simulink library "pmm"  (R2021b)
settings: Solver=VariableStepAuto  StartTime=0.0  StopTime=10.0  RelTol=1e-3
undefined symbols (not defined in the file): APMM_CoolgFanActCurr_X_pct, APMM_EWP1Curr_X_c, APMM_EWP3Curr_X_c, APMM_LVBattChktime_X_enum, APMM_LVBattChrgtime_X_enum, APMM_LVChrgLv_X_mV, ENUM_ANTITHEFT_ALARM, ENUM_ANTITHEFT_ARM, ENUM_ANTITHEFT_DISARM, ENUM_ANTITHEFT_WAIT, ENUM_APSSYSTEMSTA_REMOTEACTIVE, ENUM_CHRGPLUGSTA_NONE, ENUM_CRASHSTATE_FRONTFIRSTLV, ENUM_CRASHSTATE_LEFTSIDE, ENUM_CRASHSTATE_RIGHTSIDE, ENUM_DRIVETRAIN_AWD, ENUM_DRIVETRAIN_FWD, ENUM_DRIVETRAIN_RWD, ENUM_DRSEATSTA_EMPTY, ENUM_DRSEATSTA_INVALID, ENUM_DRSEATSTA_OCCUPIED, ENUM_EPBSTA_APPLIED, ENUM_GEARACTUALPOSN_D, ENUM_GEARACTUALPOSN_N, ENUM_GEARACTUALPOSN_P, ENUM_GEARACTUALPOSN_R, ENUM_HVBATTREADYPRE_READY, ENUM_OTACHKSTA_NOREQUEST, ENUM_OTACHKSTA_NOTIMEOUT, ENUM_OTACHKSTA_TIMEOUT, ENUM_PDKEYRAWLULOCK_INLOCK, ENUM_PDKEYRAWLULOCK_INUNLOCK, ENUM_PDKEYRAWPS_INPS, ENUM_PDKEYSTA_LOCK, ENUM_PDKEYSTA_PS, ENUM_PDKEYSTA_UNAVALIABLE, ENUM_PDKEYSTA_UNLOCK, ENUM_POWERSTA_OFF, ENUM_POWERSTA_OFFC, ENUM_POWERSTA_STANDBY, ENUM_PWRREQOTA_NOREQUEST, ENUM_PWRREQOTA_REQPOWEROFF, ENUM_PWRREQOTA_REQPOWERSTDBY, ENUM_PWRSTASW_READY, ENUM_V2LSTA_NOPLUG, ENUM_VEHICLETYPE_D31L24, ENUM_VEHMALFUNLEVEL_LEVEL3, ENUM_VEHMALFUNLEVEL_LEVEL4, FALSE, KPMM_AllDoorClosedHoldTime_s, KPMM_APSAllowThd_pct, KPMM_BattDownFailtime_s, KPMM_BattUpFailtime_s, KPMM_BattUpResetRty_cnt, KPMM_BattUpResetSW_flg, KPMM_BattUpResetTO_s, KPMM_BattUpRstDlyTO_s, KPMM_BrakeSWHoldTime_s, KPMM_CANValidChkFailtime_s, KPMM_ChrgPlugHoldTime_s ... (+87)
libraries: simulink x29, hcu_lib x24
(part 3 of 7)

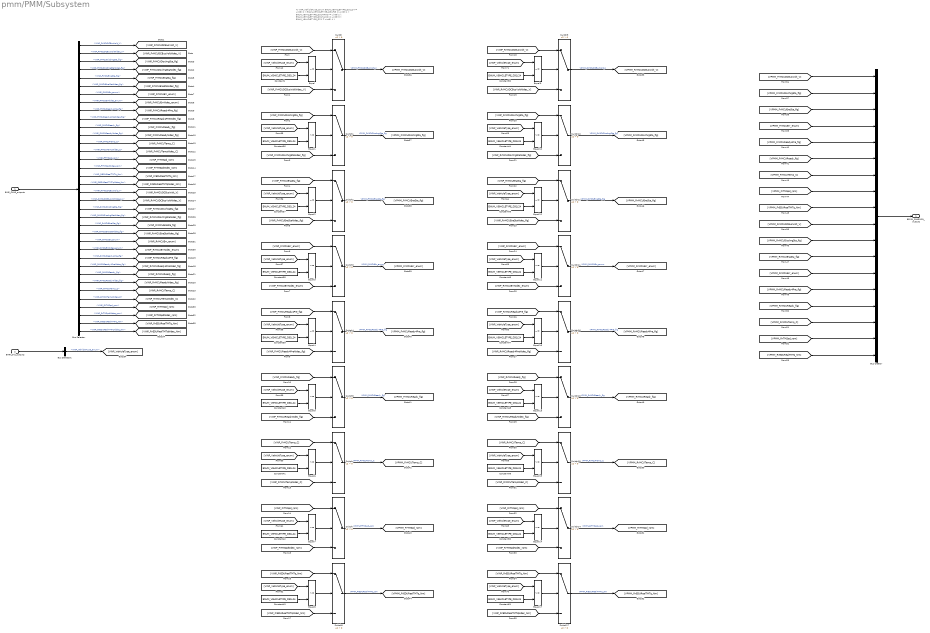
== system pmm/PMM/Subsystem ==
  note: % VINP_VehicleType_enum
      | ENUM_VEHICLETYPE_D31L24         	= uint8(  0  );
      | ENUM_VEHICLETYPE_D31F25         	= uint8(  1  );
      | ENUM_VEHICLETYPE_D31HRWD        = uint8(  2  );
      | ENUM_VEHICLETYPE_D31HAWD        = uint8(  3  );
      | ENUM_VEHICLETYPE_D21           		= uint8(  4  );
  BINP_CAN3_outputs : Inport
  BINP_SYS_outputs : Inport  Port=2
  Bus Creator : BusCreator  Inputs=18
  Bus Selector : BusSelector  OutputSignals=VINP_FrMCUDCBusVolt_V,VINP_FrMCUDCBusVoltNidec_V,VINP_FrMCUDischrgSta_flg,VINP_FrMCUDischrgStaNidec_flg,VINP_FrMCUEnaSta_flg,VINP_FrMCUEnaStaNidec_flg,VINP_FrMCUErr_enum,VINP_FrMCUErrNidec_enum,VINP_FrMCUReady4Pre_flg,VINP_FrMCUReady4PreNidec_flg,VINP_FrMCUReady_flg,VINP_FrMCUReadyNidec_flg,VINP_FrMCUTemp_C,VINP_FrMCUTempNidec_C,VINP_FrTMSpd_rpm,VINP_FrTMSpdNidec_rpm,VINP_FrEDURealTMTq_Nm,VINP_FrEDURealTMTqNidec_Nm,VINP_RrMCUDCBusVolt_V,VINP_RrMCUDCBusVoltNidec_V,VINP_RrMCUDischrgSta_flg,VINP_RrMCUDischrgStaNidec_flg,VINP_RrMCUEnaSta_flg,VINP_RrMCUEnaStaNidec_flg,VINP_RrMCUErr_enum,VINP_RrMCUErrNidec_enum,VINP_RrMCUReady4Pre_flg,VINP_RrMCUReady4PreNidec_flg,VINP_RrMCUReady_flg,VINP_RrMCUReadyNidec_flg,VINP_RrMCUTemp_C,VINP_RrMCUTempNidec_C,VINP_RrTMSpd_rpm,VINP_RrTMSpdNidec_rpm,VINP_RrEDURealTMTq_Nm,VINP_RrEDURealTMTqNidec_Nm
  Bus Selector1 : BusSelector  OutputSignals=VINP_VehicleType_enum
  Constant{1,36..52} (18 alike) : Constant  Value=ENUM_VEHICLETYPE_D31L24
  Equal{,1..17} (18 alike) : RelationalOperator  Operator=~=  OutDataTypeStr=boolean  RndMeth=Simplest
  Switch{,1..17} (18 alike) : Switch  Criteria=u2 > Threshold
  BPMM_CAN3MCU_outputs : Outport
  wires:
  BINP_CAN3_outputs/1 -> Bus Selector/1
  Bus Selector/1 -> [VINP_FrMCUDCBusVolt_V]  "<VINP_FrMCUDCBusVolt_V>"
  Bus Selector/2 -> [VINP_FrMCUDCBusVoltNidec_V]  "<VINP_FrMCUDCBusVoltNidec_V>"
  Bus Selector/3 -> [VINP_FrMCUDischrgSta_flg]  "<VINP_FrMCUDischrgSta_flg>"
  Bus Selector/4 -> [VINP_FrMCUDischrgStaNidec_flg]  "<VINP_FrMCUDischrgStaNidec_flg>"
  Bus Selector/5 -> [VINP_FrMCUEnaSta_flg]  "<VINP_FrMCUEnaSta_flg>"
  Bus Selector/6 -> [VINP_FrMCUEnaStaNidec_flg]  "<VINP_FrMCUEnaStaNidec_flg>"
  Bus Selector/7 -> [VINP_FrMCUErr_enum]  "<VINP_FrMCUErr_enum>"
  Bus Selector/8 -> [VINP_FrMCUErrNidec_enum]  "<VINP_FrMCUErrNidec_enum>"
  Bus Selector/9 -> [VINP_FrMCUReady4Pre_flg]  "<VINP_FrMCUReady4Pre_flg>"
  Bus Selector/10 -> [VINP_FrMCUReady4PreNidec_flg]  "<VINP_FrMCUReady4PreNidec_flg>"
  Bus Selector/11 -> [VINP_FrMCUReady_flg]  "<VINP_FrMCUReady_flg>"
  Bus Selector/12 -> [VINP_FrMCUReadyNidec_flg]  "<VINP_FrMCUReadyNidec_flg>"
  Bus Selector/13 -> [VINP_FrMCUTemp_C]  "<VINP_FrMCUTemp_C>"
  Bus Selector/14 -> [VINP_FrMCUTempNidec_C]  "<VINP_FrMCUTempNidec_C>"
  Bus Selector/15 -> [VINP_FrTMSpd_rpm]  "<VINP_FrTMSpd_rpm>"
  Bus Selector/16 -> [VINP_FrTMSpdNidec_rpm]  "<VINP_FrTMSpdNidec_rpm>"
  Bus Selector/17 -> [VINP_FrEDURealTMTq_Nm]  "<VINP_FrEDURealTMTq_Nm>"
  Bus Selector/18 -> [VINP_FrEDURealTMTqNidec_Nm]  "<VINP_FrEDURealTMTqNidec_Nm>"
  Bus Selector/19 -> [VINP_RrMCUDCBusVolt_V]  "<VINP_RrMCUDCBusVolt_V>"
  Bus Selector/20 -> [VINP_RrMCUDCBusVoltNidec_V]  "<VINP_RrMCUDCBusVoltNidec_V>"
  Bus Selector/21 -> [VINP_RrMCUDischrgSta_flg]  "<VINP_RrMCUDischrgSta_flg>"
  Bus Selector/22 -> [VINP_RrMCUDischrgStaNidec_flg]  "<VINP_RrMCUDischrgStaNidec_flg>"
  Bus Selector/23 -> [VINP_RrMCUEnaSta_flg]  "<VINP_RrMCUEnaSta_flg>"
  Bus Selector/24 -> [VINP_RrMCUEnaStaNidec_flg]  "<VINP_RrMCUEnaStaNidec_flg>"
  Bus Selector/25 -> [VINP_RrMCUErr_enum]  "<VINP_RrMCUErr_enum>"
  Bus Selector/26 -> [VINP_RrMCUErrNidec_enum]  "<VINP_RrMCUErrNidec_enum>"
  Bus Selector/27 -> [VINP_RrMCUReady4Pre_flg]  "<VINP_RrMCUReady4Pre_flg>"
  Bus Selector/28 -> [VINP_RrMCUReady4PreNidec_flg]  "<VINP_RrMCUReady4PreNidec_flg>"
  Bus Selector/29 -> [VINP_RrMCUReady_flg]  "<VINP_RrMCUReady_flg>"
  Bus Selector/30 -> [VINP_RrMCUReadyNidec_flg]  "<VINP_RrMCUReadyNidec_flg>"
  Bus Selector/31 -> [VINP_RrMCUTemp_C]  "<VINP_RrMCUTemp_C>"
  Bus Selector/32 -> [VINP_RrMCUTempNidec_C]  "<VINP_RrMCUTempNidec_C>"
  Bus Selector/33 -> [VINP_RrTMSpd_rpm]  "<VINP_RrTMSpd_rpm>"
  Bus Selector/34 -> [VINP_RrTMSpdNidec_rpm]  "<VINP_RrTMSpdNidec_rpm>"
  Bus Selector/35 -> [VINP_RrEDURealTMTq_Nm]  "<VINP_RrEDURealTMTq_Nm>"
  Bus Selector/36 -> [VINP_RrEDURealTMTqNidec_Nm]  "<VINP_RrEDURealTMTqNidec_Nm>"
  Constant1/1 -> Equal/2
  Equal/1 -> Switch/2
  [VINP_FrMCUDCBusVolt_V] -> Switch/1
  [VINP_FrMCUDCBusVoltNidec_V] -> Switch/3
  Switch/1 -> [VPMM_FrMCUDCBusVolt_V]  "VPMM_FrMCUDCBusVolt_V"
  Equal1/1 -> Switch1/2
  Equal2/1 -> Switch2/2
  [VINP_FrMCUEnaStaNidec_flg] -> Switch2/3
  [VINP_FrMCUEnaSta_flg] -> Switch2/1
  [VINP_FrMCUDischrgStaNidec_flg] -> Switch1/3
  [VINP_FrMCUDischrgSta_flg] -> Switch1/1
  Equal3/1 -> Switch3/2
  [VINP_FrMCUErr_enum] -> Switch3/1
  [VINP_FrMCUErrNidec_enum] -> Switch3/3
  Equal4/1 -> Switch4/2
  [VINP_FrMCUReady4Pre_flg] -> Switch4/1
  [VINP_FrMCUReady4PreNidec_flg] -> Switch4/3
  Equal5/1 -> Switch5/2
  [VINP_FrMCUReady_flg] -> Switch5/1
  [VINP_FrMCUReadyNidec_flg] -> Switch5/3
  Equal6/1 -> Switch6/2
  [VINP_FrMCUTemp_C] -> Switch6/1
  [VINP_FrMCUTempNidec_C] -> Switch6/3
  Equal7/1 -> Switch7/2
  Equal8/1 -> Switch8/2
  [VINP_FrTMSpd_rpm] -> Switch7/1
  [VINP_FrTMSpdNidec_rpm] -> Switch7/3
  [VINP_FrEDURealTMTq_Nm] -> Switch8/1
  [VINP_FrEDURealTMTqNidec_Nm] -> Switch8/3
  Equal9/1 -> Switch9/2
  Equal10/1 -> Switch10/2
  Equal11/1 -> Switch11/2
  Equal12/1 -> Switch12/2
  Equal15/1 -> Switch15/2
  Equal14/1 -> Switch14/2
  Equal13/1 -> Switch13/2
  Equal16/1 -> Switch16/2
  Equal17/1 -> Switch17/2
  [VINP_RrMCUDCBusVolt_V] -> Switch9/1
  [VINP_RrMCUDCBusVoltNidec_V] -> Switch9/3
  [VINP_RrMCUDischrgSta_flg] -> Switch10/1
  [VINP_RrMCUDischrgStaNidec_flg] -> Switch10/3
  [VINP_RrMCUEnaSta_flg] -> Switch12/1
  [VINP_RrMCUEnaStaNidec_flg] -> Switch12/3
  [VINP_RrMCUErr_enum] -> Switch11/1
  [VINP_RrMCUErrNidec_enum] -> Switch11/3
  [VINP_RrMCUReady4Pre_flg] -> Switch16/1
  [VINP_RrMCUReady4PreNidec_flg] -> Switch16/3
  [VINP_RrMCUReady_flg] -> Switch13/1
  [VINP_RrMCUReadyNidec_flg] -> Switch13/3
  [VINP_RrMCUTemp_C] -> Switch15/1
  [VINP_RrMCUTempNidec_C] -> Switch15/3
  [VINP_RrTMSpd_rpm] -> Switch14/1
  [VINP_RrTMSpdNidec_rpm] -> Switch14/3
  [VINP_RrEDURealTMTqNidec_Nm] -> Switch17/3
  [VINP_RrEDURealTMTq_Nm] -> Switch17/1
  Switch1/1 -> [VPMM_FrMCUDischrgSta_flg]  "VPMM_FrMCUDischrgSta_flg"
  Switch2/1 -> [VPMM_FrMCUEnaSta_flg]  "VPMM_FrMCUEnaSta_flg"
  Switch3/1 -> [VPMM_FrMCUErr_enum]  "VPMM_FrMCUErr_enum"
  Switch4/1 -> [VPMM_FrMCUReady4Pre_flg]  "VPMM_FrMCUReady4Pre_flg"
  Switch5/1 -> [VPMM_FrMCUReady_flg]  "VPMM_FrMCUReady_flg"
  Switch6/1 -> [VPMM_FrMCUTemp_C]  "VPMM_FrMCUTemp_C"
  Switch7/1 -> [VPMM_FrTMSpd_rpm]  "VPMM_FrTMSpd_rpm"
  Switch8/1 -> [VPMM_FrEDURealTMTq_Nm]  "VPMM_FrEDURealTMTq_Nm"
  Switch9/1 -> [VPMM_RrMCUDCBusVolt_V]  "VPMM_RrMCUDCBusVolt_V"
  Switch10/1 -> [VPMM_RrMCUDischrgSta_flg]  "VPMM_RrMCUDischrgSta_flg"
  Switch12/1 -> [VPMM_RrMCUEnaSta_flg]  "VPMM_RrMCUEnaSta_flg"
  Switch11/1 -> [VPMM_RrMCUErr_enum]  "VPMM_RrMCUErr_enum"
  Switch16/1 -> [VPMM_RrMCUReady4Pre_flg]  "VPMM_RrMCUReady4Pre_flg"
  Switch13/1 -> [VPMM_RrMCUReady_flg]  "VPMM_RrMCUReady_flg"
  Switch15/1 -> [VPMM_RrMCUTemp_C]  "VPMM_RrMCUTemp_C"
  Switch14/1 -> [VPMM_RrTMSpd_rpm]  "VPMM_RrTMSpd_rpm"
  Switch17/1 -> [VPMM_RrEDURealTMTq_Nm]  "VPMM_RrEDURealTMTq_Nm"
  [VPMM_FrMCUReady_flg] -> Bus Creator/6
  [VPMM_FrMCUReady4Pre_flg] -> Bus Creator/5
  [VPMM_FrMCUTemp_C] -> Bus Creator/7
  [VPMM_FrMCUErr_enum] -> Bus Creator/4
  [VPMM_FrTMSpd_rpm] -> Bus Creator/8
  [VPMM_FrMCUEnaSta_flg] -> Bus Creator/3
  [VPMM_FrEDURealTMTq_Nm] -> Bus Creator/9
  [VPMM_FrMCUDischrgSta_flg] -> Bus Creator/2
  [VPMM_RrMCUDischrgSta_flg] -> Bus Creator/11
  [VPMM_RrMCUEnaSta_flg] -> Bus Creator/12
  [VPMM_RrMCUErr_enum] -> Bus Creator/13
  [VPMM_RrMCUReady4Pre_flg] -> Bus Creator/14
  [VPMM_RrMCUReady_flg] -> Bus Creator/15
  [VPMM_RrMCUTemp_C] -> Bus Creator/16
  [VPMM_RrTMSpd_rpm] -> Bus Creator/17
  [VPMM_RrEDURealTMTq_Nm] -> Bus Creator/18
  Bus Creator/1 -> BPMM_CAN3MCU_outputs/1
  [VPMM_FrMCUDCBusVolt_V] -> Bus Creator/1
  [VPMM_RrMCUDCBusVolt_V] -> Bus Creator/10
  BINP_SYS_outputs/1 -> Bus Selector1/1
  Bus Selector1/1 -> [VINP_VehicleType_enum]  "<VINP_VehicleType_enum>"
  [VINP_VehicleType_enum] -> Equal/1
  [VINP_VehicleType_enum] -> Equal1/1
  Constant36/1 -> Equal1/2
  [VINP_VehicleType_enum] -> Equal2/1
  Constant37/1 -> Equal2/2
  [VINP_VehicleType_enum] -> Equal3/1
  Constant38/1 -> Equal3/2
  [VINP_VehicleType_enum] -> Equal4/1
  Constant39/1 -> Equal4/2
  [VINP_VehicleType_enum] -> Equal5/1
  Constant40/1 -> Equal5/2
  [VINP_VehicleType_enum] -> Equal6/1
  Constant41/1 -> Equal6/2
  [VINP_VehicleType_enum] -> Equal7/1
  Constant42/1 -> Equal7/2
  [VINP_VehicleType_enum] -> Equal8/1
  Constant43/1 -> Equal8/2
  [VINP_VehicleType_enum] -> Equal9/1
  Constant52/1 -> Equal9/2
  [VINP_VehicleType_enum] -> Equal10/1
  Constant44/1 -> Equal10/2
  [VINP_VehicleType_enum] -> Equal12/1
  Constant45/1 -> Equal12/2
  [VINP_VehicleType_enum] -> Equal11/1
  Constant46/1 -> Equal11/2
  [VINP_VehicleType_enum] -> Equal16/1
  Constant47/1 -> Equal16/2
  [VINP_VehicleType_enum] -> Equal13/1
  Constant48/1 -> Equal13/2
  [VINP_VehicleType_enum] -> Equal15/1
  Constant49/1 -> Equal15/2
  [VINP_VehicleType_enum] -> Equal14/1
  Constant50/1 -> Equal14/2
  [VINP_VehicleType_enum] -> Equal17/1
  Constant51/1 -> Equal17/2

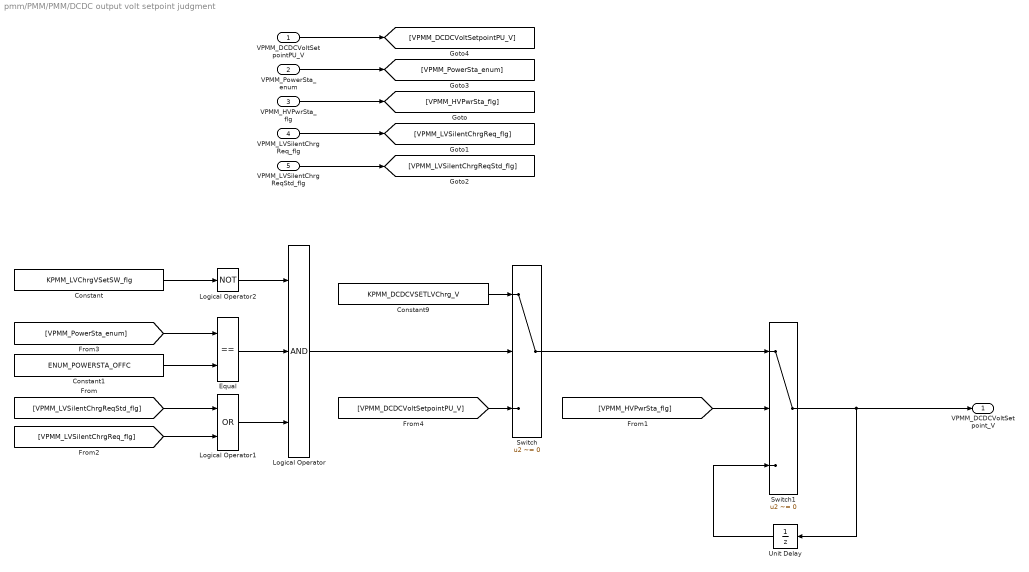
== system pmm/PMM/PMM/DCDC output volt setpoint judgment ==
  VPMM_DCDCVoltSetpointPU_V : Inport
  VPMM_PowerSta_enum : Inport  Port=2
  VPMM_HVPwrSta_flg : Inport  Port=3
  VPMM_LVSilentChrgReq_flg : Inport  Port=4
  VPMM_LVSilentChrgReqStd_flg : Inport  Port=5
  Constant : Constant  Value=KPMM_LVChrgVSetSW_flg
  Constant1 : Constant  Value=ENUM_POWERSTA_OFFC
  Constant9 : Constant  Value=KPMM_DCDCVSETLVChrg_V
  Equal : RelationalOperator  Operator===  OutDataTypeStr=boolean  RndMeth=Simplest
  Logical Operator : Logic  Inputs=3  AllPortsSameDT=off  OutDataTypeStr=boolean
  Logical Operator1 : Logic  Operator=OR  AllPortsSameDT=off  OutDataTypeStr=boolean
  Logical Operator2 : Logic  Operator=NOT  AllPortsSameDT=off  OutDataTypeStr=boolean
  Switch : Switch  Criteria=u2 ~= 0
  Switch1 : Switch  Criteria=u2 ~= 0
  Unit Delay : UnitDelay  SampleTime=-1  HasFrameUpgradeWarning=on
  VPMM_DCDCVoltSetpoint_V : Outport
  wires:
  Switch1/1 -> VPMM_DCDCVoltSetpoint_V/1, Unit Delay/1
  VPMM_PowerSta_enum/1 -> [VPMM_PowerSta_enum]
  VPMM_HVPwrSta_flg/1 -> [VPMM_HVPwrSta_flg]
  VPMM_LVSilentChrgReq_flg/1 -> [VPMM_LVSilentChrgReq_flg]
  VPMM_LVSilentChrgReqStd_flg/1 -> [VPMM_LVSilentChrgReqStd_flg]
  VPMM_DCDCVoltSetpointPU_V/1 -> [VPMM_DCDCVoltSetpointPU_V]
  Constant9/1 -> Switch/1
  Equal/1 -> Logical Operator/2
  Unit Delay/1 -> Switch1/3
  Switch/1 -> Switch1/1
  Logical Operator/1 -> Switch/2
  [VPMM_LVSilentChrgReq_flg] -> Logical Operator1/2
  [VPMM_LVSilentChrgReqStd_flg] -> Logical Operator1/1
  Logical Operator1/1 -> Logical Operator/3
  [VPMM_HVPwrSta_flg] -> Switch1/2
  Constant1/1 -> Equal/2
  [VPMM_PowerSta_enum] -> Equal/1
  [VPMM_DCDCVoltSetpointPU_V] -> Switch/3
  Logical Operator2/1 -> Logical Operator/1
  Constant/1 -> Logical Operator2/1

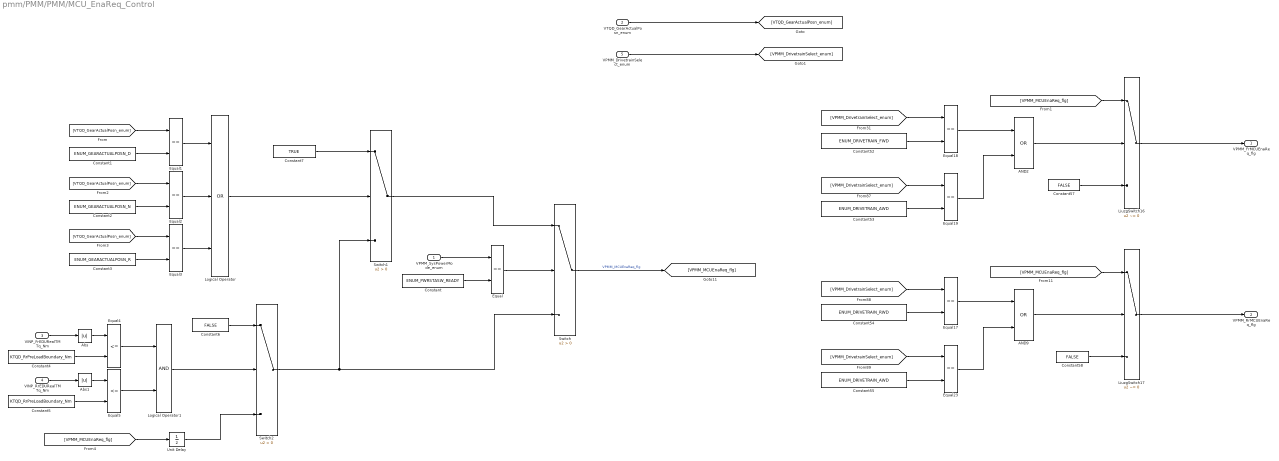
== system pmm/PMM/PMM/MCU_EnaReq_Control ==
  VPMM_SysPowerMode_enum : Inport
  VTQD_GearActualPosn_enum : Inport  Port=2
  VINP_FrEDURealTMTq_Nm : Inport  Port=3
  VINP_RrEDURealTMTq_Nm : Inport  Port=4
  VPMM_DrivetrainSelect_enum : Inport  Port=5
  AND2 : Logic  Operator=OR  AllPortsSameDT=off  OutDataTypeStr=boolean
  AND9 : Logic  Operator=OR  AllPortsSameDT=off  OutDataTypeStr=boolean
  Abs : Abs
  Abs1 : Abs
  Constant : Constant  Value=ENUM_PWRSTASW_READY
  Constant1 : Constant  Value=ENUM_GEARACTUALPOSN_D
  Constant2 : Constant  Value=ENUM_GEARACTUALPOSN_N
  Constant3 : Constant  Value=ENUM_GEARACTUALPOSN_R
  Constant4 : Constant  Value=KTQD_RrPreLoadBoundary_Nm
  Constant5 : Constant  Value=KTQD_RrPreLoadBoundary_Nm
  Constant52 : Constant  Value=ENUM_DRIVETRAIN_FWD
  Constant53 : Constant  Value=ENUM_DRIVETRAIN_AWD
  Constant54 : Constant  Value=ENUM_DRIVETRAIN_RWD
  Constant55 : Constant  Value=ENUM_DRIVETRAIN_AWD
  Constant57 : Constant  Value=FALSE
  Constant58 : Constant  Value=FALSE
  Constant6 : Constant  Value=FALSE
  Constant7 : Constant  Value=TRUE
  Equal{,1..3,17..19,23} (8 alike) : RelationalOperator  Operator===  OutDataTypeStr=boolean  RndMeth=Simplest
  Equal4 : RelationalOperator  Operator=<=  OutDataTypeStr=boolean  RndMeth=Simplest
  Equal5 : RelationalOperator  Operator=<=  OutDataTypeStr=boolean  RndMeth=Simplest
  LiuzgSwitch16 : Switch  Criteria=u2 ~= 0
      settings: AttributesFormatString=<%<Criteria>>
  LiuzgSwitch17 : Switch  Criteria=u2 ~= 0
      settings: AttributesFormatString=<%<Criteria>>
  Logical Operator : Logic  Operator=OR  Inputs=3  AllPortsSameDT=off  OutDataTypeStr=boolean
  Logical Operator1 : Logic  AllPortsSameDT=off  OutDataTypeStr=boolean
  Switch : Switch  Criteria=u2 > Threshold
  Switch1 : Switch  Criteria=u2 > Threshold
  Switch2 : Switch  Criteria=u2 > Threshold
  Unit Delay : UnitDelay  SampleTime=-1  HasFrameUpgradeWarning=on
  VPMM_FrMCUEnaReq_flg : Outport
  VPMM_RrMCUEnaReq_flg : Outport  Port=2
  wires:
  VPMM_DrivetrainSelect_enum/1 -> [VPMM_DrivetrainSelect_enum]
  LiuzgSwitch17/1 -> VPMM_RrMCUEnaReq_flg/1
  Constant57/1 -> LiuzgSwitch16/3
  [VPMM_DrivetrainSelect_enum] -> Equal19/1
  Constant55/1 -> Equal23/2
  Constant58/1 -> LiuzgSwitch17/3
  Constant54/1 -> Equal17/2
  Constant53/1 -> Equal19/2
  Equal19/1 -> AND2/2
  [VPMM_DrivetrainSelect_enum] -> Equal17/1
  [VPMM_MCUEnaReq_flg] -> LiuzgSwitch16/1
  [VPMM_MCUEnaReq_flg] -> LiuzgSwitch17/1
  AND2/1 -> LiuzgSwitch16/2
  [VPMM_DrivetrainSelect_enum] -> Equal23/1
  Equal17/1 -> AND9/1
  Constant52/1 -> Equal18/2
  [VPMM_DrivetrainSelect_enum] -> Equal18/1
  Equal18/1 -> AND2/1
  LiuzgSwitch16/1 -> VPMM_FrMCUEnaReq_flg/1
  AND9/1 -> LiuzgSwitch17/2
  Equal23/1 -> AND9/2
  VPMM_SysPowerMode_enum/1 -> Equal/1
  Constant/1 -> Equal/2
  Equal/1 -> Switch/2
  Switch1/1 -> Switch/1
  Switch/1 -> [VPMM_MCUEnaReq_flg]  "VPMM_MCUEnaReq_flg"
  VTQD_GearActualPosn_enum/1 -> [VTQD_GearActualPosn_enum]
  [VTQD_GearActualPosn_enum] -> Equal1/1
  [VTQD_GearActualPosn_enum] -> Equal2/1
  [VTQD_GearActualPosn_enum] -> Equal3/1
  Constant3/1 -> Equal3/2
  Constant2/1 -> Equal2/2
  Constant1/1 -> Equal1/2
  Equal3/1 -> Logical Operator/3
  Equal2/1 -> Logical Operator/2
  Equal1/1 -> Logical Operator/1
  Logical Operator/1 -> Switch1/2
  Switch2/1 -> Switch1/3, Switch/3
  Equal4/1 -> Logical Operator1/1
  Equal5/1 -> Logical Operator1/2
  Logical Operator1/1 -> Switch2/2
  VINP_FrEDURealTMTq_Nm/1 -> Abs/1
  VINP_RrEDURealTMTq_Nm/1 -> Abs1/1
  Constant4/1 -> Equal4/2
  Constant5/1 -> Equal5/2
  [VPMM_MCUEnaReq_flg] -> Unit Delay/1
  Unit Delay/1 -> Switch2/3
  Constant6/1 -> Switch2/1
  Constant7/1 -> Switch1/1
  Abs/1 -> Equal4/1
  Abs1/1 -> Equal5/1

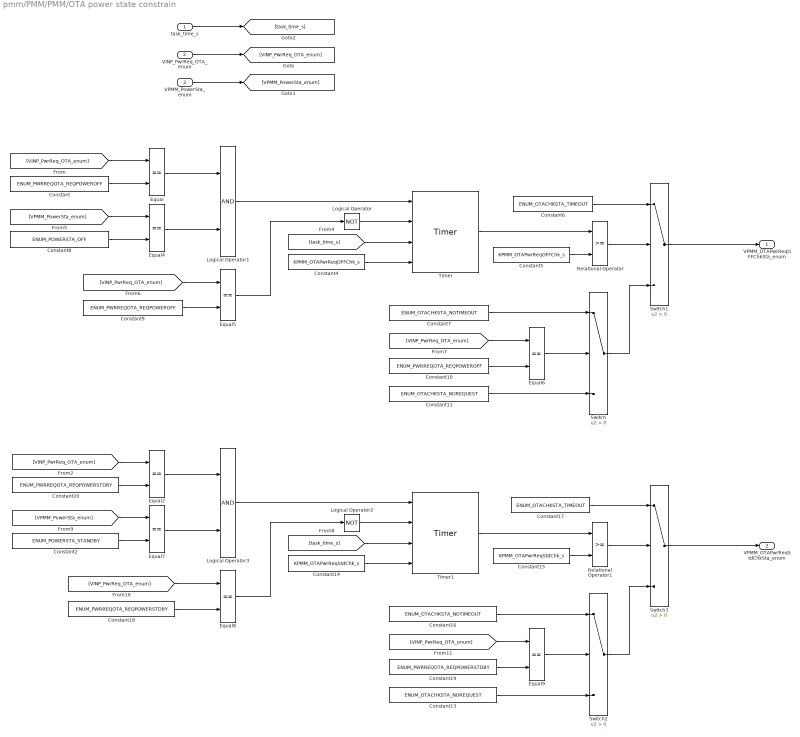
== system pmm/PMM/PMM/OTA power state constrain ==
  task_time_s : Inport
  VINP_PwrReq_OTA_enum : Inport  Port=2
  VPMM_PowerSta_enum : Inport  Port=3
  Constant : Constant  Value=ENUM_PWRREQOTA_REQPOWEROFF
  Constant10 : Constant  Value=ENUM_PWRREQOTA_REQPOWEROFF
  Constant11 : Constant  Value=ENUM_OTACHKSTA_NOREQUEST
  Constant13 : Constant  Value=ENUM_OTACHKSTA_NOREQUEST
  Constant14 : Constant  Value=KPMM_OTAPwrReqStdChk_s
  Constant15 : Constant  Value=KPMM_OTAPwrReqStdChk_s
  Constant16 : Constant  Value=ENUM_OTACHKSTA_NOTIMEOUT
  Constant17 : Constant  Value=ENUM_OTACHKSTA_TIMEOUT
  Constant18 : Constant  Value=ENUM_PWRREQOTA_REQPOWERSTDBY
  Constant19 : Constant  Value=ENUM_PWRREQOTA_REQPOWERSTDBY
  Constant2 : Constant  Value=ENUM_POWERSTA_STANDBY
  Constant20 : Constant  Value=ENUM_PWRREQOTA_REQPOWERSTDBY
  Constant4 : Constant  Value=KPMM_OTAPwrReqOFFChk_s
  Constant5 : Constant  Value=KPMM_OTAPwrReqOFFChk_s
  Constant6 : Constant  Value=ENUM_OTACHKSTA_TIMEOUT
  Constant7 : Constant  Value=ENUM_OTACHKSTA_NOTIMEOUT
  Constant8 : Constant  Value=ENUM_POWERSTA_OFF
  Constant9 : Constant  Value=ENUM_PWRREQOTA_REQPOWEROFF
  Equal{,2,4..9} (8 alike) : RelationalOperator  Operator===  OutDataTypeStr=boolean  RndMeth=Simplest
  Logical Operator : Logic  Operator=NOT  AllPortsSameDT=off  OutDataTypeStr=boolean
  Logical Operator1 : Logic  AllPortsSameDT=off  OutDataTypeStr=boolean
  Logical Operator2 : Logic  Operator=NOT  AllPortsSameDT=off  OutDataTypeStr=boolean
  Logical Operator3 : Logic  AllPortsSameDT=off  OutDataTypeStr=boolean
  Relational Operator : RelationalOperator  OutDataTypeStr=boolean  RndMeth=Simplest
  Relational Operator1 : RelationalOperator  OutDataTypeStr=boolean  RndMeth=Simplest
  Switch{,1..3} (4 alike) : Switch  Criteria=u2 > Threshold
  Timer : hcu_lib/Basic_Blocks/Timer
  Timer1 : hcu_lib/Basic_Blocks/Timer
  VPMM_OTAPwrReqOFFChkSta_enum : Outport
  VPMM_OTAPwrReqStdChkSta_enum : Outport  Port=2
  wires:
  Constant/1 -> Equal/2
  VINP_PwrReq_OTA_enum/1 -> [VINP_PwrReq_OTA_enum]
  VPMM_PowerSta_enum/1 -> [VPMM_PowerSta_enum]
  [VINP_PwrReq_OTA_enum] -> Equal/1
  task_time_s/1 -> [task_time_s]
  [task_time_s] -> Timer/3
  Constant4/1 -> Timer/4
  Constant5/1 -> Relational Operator/2
  Timer/1 -> Relational Operator/1
  Relational Operator/1 -> Switch1/2
  Logical Operator/1 -> Timer/2
  Constant8/1 -> Equal4/2
  [VPMM_PowerSta_enum] -> Equal4/1
  Equal/1 -> Logical Operator1/1
  Equal4/1 -> Logical Operator1/2
  Logical Operator1/1 -> Timer/1
  [VINP_PwrReq_OTA_enum] -> Equal5/1
  Constant9/1 -> Equal5/2
  Equal5/1 -> Logical Operator/1
  Constant6/1 -> Switch1/1
  Constant10/1 -> Equal6/2
  [VINP_PwrReq_OTA_enum] -> Equal6/1
  Equal6/1 -> Switch/2
  Constant7/1 -> Switch/1
  Switch/1 -> Switch1/3
  Constant11/1 -> Switch/3
  Switch1/1 -> VPMM_OTAPwrReqOFFChkSta_enum/1
  Switch2/1 -> Switch3/3
  Equal9/1 -> Switch2/2
  [VINP_PwrReq_OTA_enum] -> Equal9/1
  Equal8/1 -> Logical Operator2/1
  [VINP_PwrReq_OTA_enum] -> Equal8/1
  Logical Operator3/1 -> Timer1/1
  Equal7/1 -> Logical Operator3/2
  Equal2/1 -> Logical Operator3/1
  [VPMM_PowerSta_enum] -> Equal7/1
  Logical Operator2/1 -> Timer1/2
  Relational Operator1/1 -> Switch3/2
  Timer1/1 -> Relational Operator1/1
  Constant15/1 -> Relational Operator1/2
  Constant14/1 -> Timer1/4
  [task_time_s] -> Timer1/3
  [VINP_PwrReq_OTA_enum] -> Equal2/1
  Constant20/1 -> Equal2/2
  Constant13/1 -> Switch2/3
  Constant16/1 -> Switch2/1
  Constant17/1 -> Switch3/1
  Switch3/1 -> VPMM_OTAPwrReqStdChkSta_enum/1
  Constant2/1 -> Equal7/2
  Constant18/1 -> Equal8/2
  Constant19/1 -> Equal9/2
